simulink model "analysis3"  (Simulink 9.0)
settings: Solver=VariableStepDiscrete  StartTime=0.0  StopTime=10.0  FixedStep=5e-5  RelTol=1e-3
libraries: commanapbnd3 x2, commchan3 x1
settings Model: Creator=CQC  LastModifiedBy=CQC
settings DataIOCC: SaveFormat=Dataset
settings OptimizationCC: LifeSpan=auto
settings DebuggingCC: UnderspecifiedInitializationDetection=Simplified  MergeDetectMultiDrivingBlocksExec=error  SFUnexpectedBacktrackingDiag=error  SFNoUnconditionalDefaultTransitionDiag=error  SFExecutionAtInitializationDiag=warning
settings HardwareCC: ProdBitPerPointer=64  ProdBitPerSizeT=64  ProdBitPerPtrDiffT=64  ProdLargestAtomicFloat=Float  ProdIntDivRoundTo=Zero  ProdEndianess=LittleEndian  ProdWordSize=64  ProdHWDeviceType=Intel->x86-64 (Windows64)
settings ModelReferenceCC: PropagateSignalLabelsOutOfModel=on
settings CodeAppCC: StateflowObjectComments=off
settings GRTTargetCC: TargetLangStandard=C99 (ISO)
settings ConfigComp: CovMetricSettings=dwe  CovHtmlReporting=off  CovSaveCumulativeToWorkspaceVar=off  CovSaveSingleToWorkspaceVar=off  CovExternalEMLEnable=on

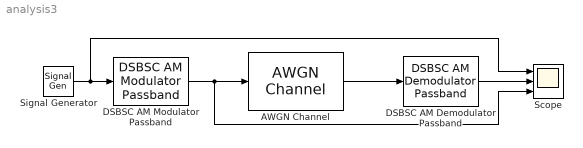
== system analysis3 ==
  AWGN Channel : commchan3/AWGN Channel  InputProcessing=Columns as channels (frame based)  seed=67  noiseMode="Signal to noise ratio  (Eb/No)"  EbNodB=10  EsNodB=10  SNRdB=10  bitsPerSym=1  Ps=0.25  Tsym=1  variance=1
  DSBSC AM Demodulator Passband : commanapbnd3/DSBSC AM Demodulator Passband  Fc=300  Ph=0  method=Butterworth  n=4  cf=300  Rp=0.1  Rs=50
      settings: SourceProductName=Communications System Toolbox  SourceProductBaseCode=CM
  DSBSC AM Modulator Passband : commanapbnd3/DSBSC AM Modulator Passband  Fc=300  Ph=0
      settings: SourceProductName=Communications System Toolbox  SourceProductBaseCode=CM
  Scope : Scope  NumInputPorts=3
  Signal Generator : SignalGenerator  Frequency=3  VectorParams1D=off
  wires:
  Signal Generator/1 -> DSBSC AM Modulator Passband/1, Scope/1
  DSBSC AM Modulator Passband/1 -> Scope/3, AWGN Channel/1
  AWGN Channel/1 -> DSBSC AM Demodulator Passband/1
  DSBSC AM Demodulator Passband/1 -> Scope/2
